simulink model "DiRe"  (Simulink 8.5)
settings: Solver=ode23t  SolverMode=SingleTasking  StartTime=0.0  StopTime=0.08  FixedStep=1e-5  MaxStep=0.7e-4  RelTol=1e-3  AbsTol=1e-2
libraries: powerlib x40, powerlib_extras x4
settings Model: Creator=azadpour  LastModifiedBy=PC
settings DataIOCC: LimitDataPoints=off
settings OptimizationCC: BlockReduction=off  BooleanDataType=off  InitFltsAndDblsToZero=on
settings DebuggingCC: SaveWithParameterizedLinksMsg=none  SignalResolutionControl=TryResolveAllWithWarning  MultiTaskDSMMsg=warning  MultiTaskCondExecSysMsg=none  FcnCallInpInsideContextMsg=UseLocalSettings
settings HardwareCC: TargetUnknown=on
settings GRTTargetCC: TargetFcnLib=ansi_tfl_tmw.mat

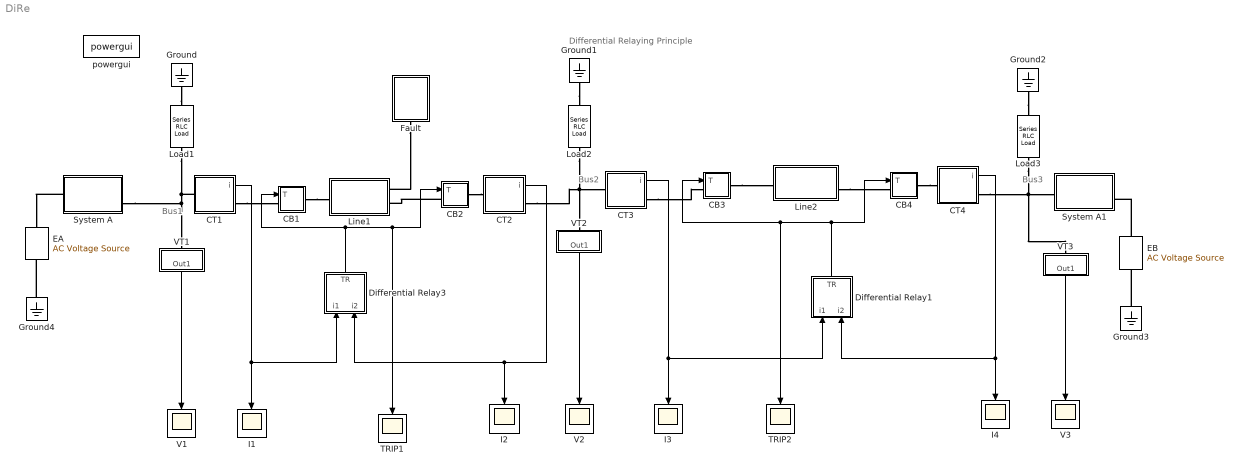
== system DiRe ==
  note: Differential Relaying Principle
  note: Bus3
  note: Bus2
  note: Bus1
  CB1 : Subsystem  mask(CB){t_op=15}
      mask prompts: t_op "Operating time [ms]"
      mask Display: disp('CB')
  CB2 : Subsystem  mask(CB){t_op=25}
      mask prompts: t_op "Operating time [ms]"
      mask Display: disp('CB')
  CB3 : Subsystem  mask(CB){t_op=18}
      mask prompts: t_op "Operating time [ms]"
      mask Display: disp('CB')
  CB4 : Subsystem  mask(CB){t_op=21}
      mask prompts: t_op "Operating time [ms]"
      mask Display: disp('CB')
  CT1 : Subsystem  mask(CT){Prim=2000, Sec=4.5}
      mask prompts: Prim "Primary Current [A]"; Sec "Secondary Current [A]"
      mask Display: disp('CT')
  CT2 : Subsystem  mask(CT){Prim=2000, Sec=1}
      mask prompts: Prim "Primary Current [A]"; Sec "Secondary Current [A]"
      mask Display: disp('CT')
  CT3 : Subsystem  mask(CT){Prim=2000, Sec=5}
      mask prompts: Prim "Primary Current [A]"; Sec "Secondary Current [A]"
      mask Display: disp('CT')
  CT4 : Subsystem  mask(CT){Prim=2000, Sec=5}
      mask prompts: Prim "Primary Current [A]"; Sec "Secondary Current [A]"
      mask Display: disp('CT')
  Differential Relay1 : Subsystem
  Differential Relay3 : Subsystem
  EA : powerlib/Electrical Sources/AC Voltage Source  Amplitude=158000  Phase=0  Frequency=60  SampleTime=0  Measurements=None
  EB : powerlib/Electrical Sources/AC Voltage Source  Amplitude=145000  Phase=-15  Frequency=60  SampleTime=0  Measurements=None
  Fault : Subsystem  mask(Fault){RF=152, tf=0.02}
      mask prompts: RF "Resistance [ohm]"; tf "Time [sec]"
      mask Display: plot(0,0,100,100,[44,47,56,38,50],[23,8,64,44,97],[56,47],[25,8])
  Ground{,1..4} (5 alike) : powerlib/Elements/Ground  LConnTagsString=a
  I{1..4} (4 alike) : Scope
      I1 settings: TickLabels=on  YMin=-20  YMax=30
      I2 settings: TickLabels=on  TimeRange=0.08  YMin=-20  YMax=30
      I3 settings: TickLabels=on  YMin=-10  YMax=20
      I4 settings: TickLabels=on  YMin=-10  YMax=20
  Line1 : Subsystem  mask(Simple Line){R=2, X=20, p=0.5}
      mask prompts: R "Resistance [ohm]"; X "Reactance [ohm]"; p "Fault location [pu]"
      mask init:
      | R1=R*p; R2=R*(1-p);
      | L1=X*p/(2*pi*60);L2=X*(1-p)/(2*pi*60);
  Line2 : Subsystem  mask(Simple Line){R=2, X=20, p=0.2}
      mask prompts: R "Resistance [ohm]"; X "Reactance [ohm]"; p "Fault location [pu]"
      mask init:
      | R1=R*p; R2=R*(1-p);
      | L1=X*p/(2*pi*60);L2=X*(1-p)/(2*pi*60);
  Load1 : powerlib/Elements/Series RLC Load  LConnTagsString=a  RConnTagsString=__new0  NominalVoltage=138e3  NominalFrequency=60  ActivePower=100e6  InductivePower=30e6  CapacitivePower=0  Setx0=off  InitialVoltage=0  SetiL0=off  InitialCurrent=0  Measurements=None
  Load2 : powerlib/Elements/Series RLC Load  LConnTagsString=a  RConnTagsString=__new0  NominalVoltage=138e3  NominalFrequency=60  ActivePower=100e6  InductivePower=30e6  CapacitivePower=0  Setx0=off  InitialVoltage=0  SetiL0=off  InitialCurrent=0  Measurements=None
  Load3 : powerlib/Elements/Series RLC Load  LConnTagsString=a  RConnTagsString=__new0  NominalVoltage=138e3  NominalFrequency=60  ActivePower=100e6  InductivePower=30e6  CapacitivePower=0  Setx0=off  InitialVoltage=0  SetiL0=off  InitialCurrent=0  Measurements=None
  System A : Subsystem  mask(Simple Line){R=1, X=10, p=0.5}
      mask prompts: R "Resistance [ohm]"; X "Reactance [ohm]"; p "Fault location [pu]"
      mask init:
      | R1=R*p; R2=R*(1-p);
      | L1=X*p/(2*pi*60);L2=X*(1-p)/(2*pi*60);
  System A1 : Subsystem  mask(Simple Line){R=1, X=10, p=0.5}
      mask prompts: R "Resistance [ohm]"; X "Reactance [ohm]"; p "Fault location [pu]"
      mask init:
      | R1=R*p; R2=R*(1-p);
      | L1=X*p/(2*pi*60);L2=X*(1-p)/(2*pi*60);
  TRIP1 : Scope
      settings: TickLabels=on  YMin=-1  YMax=2
  TRIP2 : Scope
      settings: TickLabels=on  YMin=-1  YMax=1
  V1 : Scope
      settings: TickLabels=on  YMin=-175000  YMax=175000
  V2 : Scope
      settings: TickLabels=on  YMin=-15000  YMax=15000
  V3 : Scope
      settings: TickLabels=on  YMin=-125000  YMax=125000
  VT1 : Subsystem  mask(VT){vol1=138, vol2=100}
      mask prompts: vol1 "Primary voltage [kV]"; vol2 "Secondary voltage [V]"
      mask Display: disp('VT')
  VT2 : Subsystem  mask(VT){vol1=138, vol2=100}
      mask prompts: vol1 "Primary voltage [kV]"; vol2 "Secondary voltage [V]"
      mask Display: disp('VT')
  VT3 : Subsystem  mask(VT){vol1=138, vol2=100}
      mask prompts: vol1 "Primary voltage [kV]"; vol2 "Secondary voltage [V]"
      mask Display: disp('VT')
  powergui : powerlib/powergui  SimulationMode=Continuous  SolverType=Tustin/Backward Euler (TBE)  SampleTime=0  frequency=60  SPID=off  DisableSnubberDevices=off  DisableRonSwitches=off  DisableVfSwitches=off  SwTol=0  DisplayEquations=off  Interpol=off  methode=off  Ts=0  FunctionMessages=off  echomessages=off  HookPort=off  EnableUseOfTLC=off  x0status=blocks  frequencyindice=60  Pbase=100e6  ErrMax=1e-4  Iterations=50  UnitsV=kV  UnitsW=MW  buscounter=0  RestoreLinks=warning  ResistiveCurrentMeasurement=off  Frange=[0:2:500]  Ylog=off  Xlog=on  ShowGrid=off  save=off  variable=ZData  ZoomFFT=on  StartTime=0.0  cycles=1  DisplayStyle=1  fundamental=60  FreqAxis=off  MaxFrequency=1000  frequencyindicesteady=1  RmsSteady=1  display=off
  wires:
  VT2/1(Out1) -> V2/1
  Differential Relay1/1(TR) -> CB3/1(T), TRIP2/1, CB4/1(T)
  VT1/1(Out1) -> V1/1
  CT1/1(i) -> Differential Relay3/1(i1), I1/1
  Differential Relay3/1(TR) -> CB2/1(T), TRIP1/1, CB1/1(T)
  CT3/1(i) -> I3/1, Differential Relay1/1(i1)
  CT2/1(i) -> Differential Relay3/2(i2), I2/1
  VT3/1(Out1) -> V3/1
  CT4/1(i) -> I4/1, Differential Relay1/2(i2)
  connections:
  Ground4/LConn1 -- EA/LConn1
  System A/LConn1 -- EA/RConn1
  CT1/LConn1 -- Load1/RConn1 -- VT1/LConn1 -- System A/RConn2
  Ground/LConn1 -- Load1/LConn1
  CB2/LConn1 -- Line1/RConn2
  CB1/RConn1 -- Line1/LConn1
  CT1/RConn1 -- CB1/LConn1
  CT3/RConn1 -- CB3/LConn1
  CB2/RConn1 -- CT2/LConn1
  Ground1/LConn1 -- Load2/LConn1
  CB3/RConn1 -- Line2/LConn1
  Load2/RConn1 -- VT2/LConn1 -- CT3/LConn1 -- CT2/RConn1
  Load3/RConn1 -- VT3/LConn1 -- System A1/LConn1 -- CT4/RConn1
  EB/RConn1 -- System A1/RConn2
  Ground3/LConn1 -- EB/LConn1
  CB4/RConn1 -- CT4/LConn1
  Ground2/LConn1 -- Load3/LConn1
  Line2/RConn2 -- CB4/LConn1
  Fault/LConn1 -- Line1/RConn1

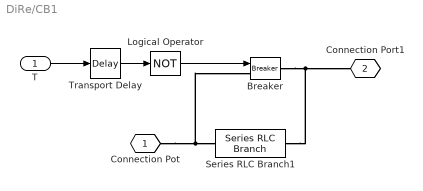
== system DiRe/CB1 ==
  T : Inport
  Breaker : powerlib/Elements/Breaker  Tag=PoWeRsYsTeMbLoCk  InitialState=1  SwitchingTimes="[ 1/60  5/60 ]"  External=on  BreakerResistance=0.01  SnubberResistance=1e6  SnubberCapacitance=inf  Measurements=None  MoreParameters=off  NoBreakLoop=off
  Logical Operator : Logic  Operator=NOT  Inputs=1
  Series RLC Branch1 : powerlib/Elements/Series RLC Branch  LConnTagsString=__new0  RConnTagsString=__new0  BranchType=R  Resistance=10000  Inductance=1.0  SetiL0=off  InitialCurrent=0  Capacitance=1.0  Setx0=off  InitialVoltage=0  Measurements=None
  Transport Delay : TransportDelay  DelayTime=t_op/1000
  Connection Pot : PMIOPort  Tag=PMCPort  Port=1  Side=Left
  Connection Port1 : PMIOPort  Tag=PMCPort  Port=2  Side=Right
  wires:
  T/1 -> Transport Delay/1
  Transport Delay/1 -> Logical Operator/1
  Logical Operator/1 -> Breaker/1
  connections:
  Connection Pot/RConn1 -- Series RLC Branch1/LConn1 -- Breaker/LConn1
  Breaker/RConn1 -- Connection Port1/RConn1 -- Series RLC Branch1/RConn1

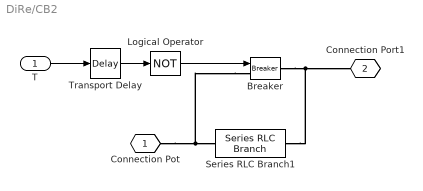
== system DiRe/CB2 ==
  T : Inport
  Breaker : powerlib/Elements/Breaker  Tag=PoWeRsYsTeMbLoCk  InitialState=1  SwitchingTimes="[ 1/60  5/60 ]"  External=on  BreakerResistance=0.01  SnubberResistance=1e6  SnubberCapacitance=inf  Measurements=None  MoreParameters=off  NoBreakLoop=off
  Logical Operator : Logic  Operator=NOT  Inputs=1
  Series RLC Branch1 : powerlib/Elements/Series RLC Branch  LConnTagsString=__new0  RConnTagsString=__new0  BranchType=R  Resistance=10000  Inductance=1e-3  SetiL0=off  InitialCurrent=0  Capacitance=1e-6  Setx0=off  InitialVoltage=0  Measurements=None
  Transport Delay : TransportDelay  DelayTime=t_op/1000
  Connection Pot : PMIOPort  Tag=PMCPort  Port=1  Side=Left
  Connection Port1 : PMIOPort  Tag=PMCPort  Port=2  Side=Right
  wires:
  Logical Operator/1 -> Breaker/1
  Transport Delay/1 -> Logical Operator/1
  T/1 -> Transport Delay/1
  connections:
  Series RLC Branch1/RConn1 -- Connection Port1/RConn1 -- Breaker/RConn1
  Breaker/LConn1 -- Series RLC Branch1/LConn1 -- Connection Pot/RConn1

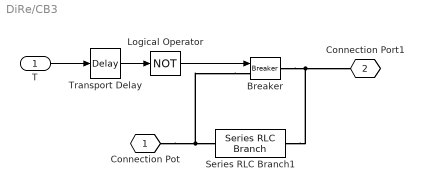
== system DiRe/CB3 ==
  T : Inport
  Breaker : powerlib/Elements/Breaker  Tag=PoWeRsYsTeMbLoCk  InitialState=1  SwitchingTimes="[ 1/60  5/60 ]"  External=on  BreakerResistance=0.01  SnubberResistance=1e6  SnubberCapacitance=inf  Measurements=None  MoreParameters=off  NoBreakLoop=off
  Logical Operator : Logic  Operator=NOT  Inputs=1
  Series RLC Branch1 : powerlib/Elements/Series RLC Branch  LConnTagsString=__new0  RConnTagsString=__new0  BranchType=R  Resistance=10000  Inductance=1e-3  SetiL0=off  InitialCurrent=0  Capacitance=1e-6  Setx0=off  InitialVoltage=0  Measurements=None
  Transport Delay : TransportDelay  DelayTime=t_op/1000
  Connection Pot : PMIOPort  Tag=PMCPort  Port=1  Side=Left
  Connection Port1 : PMIOPort  Tag=PMCPort  Port=2  Side=Right
  wires:
  Logical Operator/1 -> Breaker/1
  Transport Delay/1 -> Logical Operator/1
  T/1 -> Transport Delay/1
  connections:
  Series RLC Branch1/RConn1 -- Connection Port1/RConn1 -- Breaker/RConn1
  Breaker/LConn1 -- Series RLC Branch1/LConn1 -- Connection Pot/RConn1

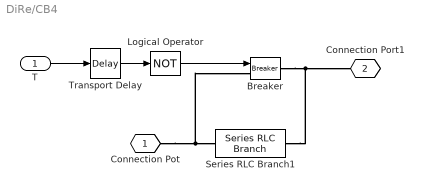
== system DiRe/CB4 ==
  T : Inport
  Breaker : powerlib/Elements/Breaker  Tag=PoWeRsYsTeMbLoCk  InitialState=1  SwitchingTimes="[ 1/60  5/60 ]"  External=on  BreakerResistance=0.01  SnubberResistance=1e6  SnubberCapacitance=inf  Measurements=None  MoreParameters=off  NoBreakLoop=off
  Logical Operator : Logic  Operator=NOT  Inputs=1
  Series RLC Branch1 : powerlib/Elements/Series RLC Branch  LConnTagsString=__new0  RConnTagsString=__new0  BranchType=R  Resistance=10000  Inductance=1e-3  SetiL0=off  InitialCurrent=0  Capacitance=1e-6  Setx0=off  InitialVoltage=0  Measurements=None
  Transport Delay : TransportDelay  DelayTime=t_op/1000
  Connection Pot : PMIOPort  Tag=PMCPort  Port=1  Side=Left
  Connection Port1 : PMIOPort  Tag=PMCPort  Port=2  Side=Right
  wires:
  T/1 -> Transport Delay/1
  Transport Delay/1 -> Logical Operator/1
  Logical Operator/1 -> Breaker/1
  connections:
  Connection Pot/RConn1 -- Series RLC Branch1/LConn1 -- Breaker/LConn1
  Breaker/RConn1 -- Connection Port1/RConn1 -- Series RLC Branch1/RConn1

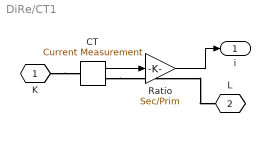
== system DiRe/CT1 ==
  CT : powerlib/Measurements/Current Measurement  PhasorSimulation=off  OutputType=Complex  PSBequivalent=0
  Ratio : Gain  Gain=Sec/Prim  SaturateOnIntegerOverflow=on  OutDataTypeStr=Inherit: Same as input  ParamDataTypeStr=Inherit: Same as input
  K : PMIOPort  Tag=PMCPort  Port=1  Side=Left
  L : PMIOPort  Tag=PMCPort  Port=2  Side=Right
  i : Outport  InitialOutput=0
  wires:
  CT/1 -> Ratio/1
  Ratio/1 -> i/1
  connections:
  K/RConn1 -- CT/LConn1
  CT/RConn1 -- L/RConn1

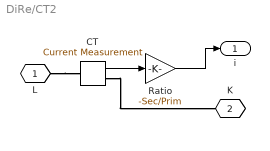
== system DiRe/CT2 ==
  CT : powerlib/Measurements/Current Measurement  PhasorSimulation=off  OutputType=Complex  PSBequivalent=0
  Ratio : Gain  Gain=-Sec/Prim  SaturateOnIntegerOverflow=on  OutDataTypeStr=Inherit: Same as input  ParamDataTypeStr=Inherit: Same as input
  L : PMIOPort  Tag=PMCPort  Port=1  Side=Left
  K : PMIOPort  Tag=PMCPort  Port=2  Side=Right
  i : Outport  InitialOutput=0
  wires:
  Ratio/1 -> i/1
  CT/1 -> Ratio/1
  connections:
  CT/RConn1 -- K/RConn1
  L/RConn1 -- CT/LConn1

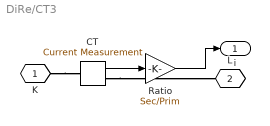
== system DiRe/CT3 ==
  CT : powerlib/Measurements/Current Measurement  PhasorSimulation=off  OutputType=Complex  PSBequivalent=0
  Ratio : Gain  Gain=Sec/Prim  SaturateOnIntegerOverflow=on  OutDataTypeStr=Inherit: Same as input  ParamDataTypeStr=Inherit: Same as input
  K : PMIOPort  Tag=PMCPort  Port=1  Side=Left
  L : PMIOPort  Tag=PMCPort  Port=2  Side=Right
  i : Outport  InitialOutput=0
  wires:
  Ratio/1 -> i/1
  CT/1 -> Ratio/1
  connections:
  CT/RConn1 -- L/RConn1
  K/RConn1 -- CT/LConn1

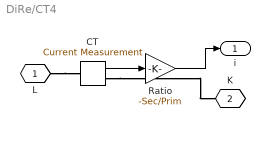
== system DiRe/CT4 ==
  CT : powerlib/Measurements/Current Measurement  PhasorSimulation=off  OutputType=Complex  PSBequivalent=0
  Ratio : Gain  Gain=-Sec/Prim  SaturateOnIntegerOverflow=on  OutDataTypeStr=Inherit: Same as input  ParamDataTypeStr=Inherit: Same as input
  L : PMIOPort  Tag=PMCPort  Port=1  Side=Left
  K : PMIOPort  Tag=PMCPort  Port=2  Side=Right
  i : Outport  InitialOutput=0
  wires:
  CT/1 -> Ratio/1
  Ratio/1 -> i/1
  connections:
  L/RConn1 -- CT/LConn1
  CT/RConn1 -- K/RConn1

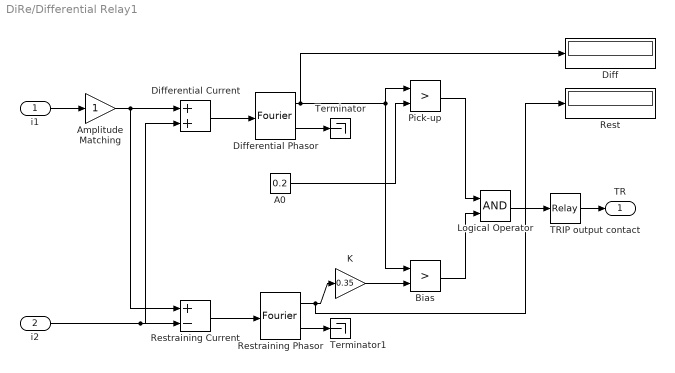
== system DiRe/Differential Relay1 ==
  i1 : Inport
  i2 : Inport  Port=2
  A0 : Constant  Value=0.2
  Amplitude Matching : Gain  SaturateOnIntegerOverflow=on  OutDataTypeStr=Inherit: Same as input  ParamDataTypeStr=Inherit: Same as input
  Bias : RelationalOperator  Operator=>  InputSameDT=on
  Diff : Display
  Differential Current : Sum  SaturateOnIntegerOverflow=on  InputSameDT=on  OutDataTypeStr=Inherit: Same as first input
  Differential Phasor : powerlib_extras/Measurements/Fourier  f1=60  n=1
  K : Gain  Gain=0.35  SaturateOnIntegerOverflow=on  OutDataTypeStr=Inherit: Same as input  ParamDataTypeStr=Inherit: Same as input
  Logical Operator : Logic
  Pick-up : RelationalOperator  Operator=>  InputSameDT=on
  Rest : Display
  Restraining Current : Sum  Inputs=+-  SaturateOnIntegerOverflow=on  InputSameDT=on  OutDataTypeStr=Inherit: Same as first input
  Restraining Phasor : powerlib_extras/Measurements/Fourier  f1=60  n=1
  TRIP output contact : Relay  OnSwitchValue=0.9999  OffSwitchValue=-1
  Terminator : Terminator
  Terminator1 : Terminator
  TR : Outport  InitialOutput=0
  wires:
  i1/1 -> Amplitude Matching/1
  Amplitude Matching/1 -> Differential Current/1, Restraining Current/1
  Differential Phasor/2 -> Terminator/1
  i2/1 -> Differential Current/2, Restraining Current/2
  Restraining Current/1 -> Restraining Phasor/1
  Restraining Phasor/2 -> Terminator1/1
  K/1 -> Bias/2
  A0/1 -> Pick-up/2
  Differential Current/1 -> Differential Phasor/1
  Bias/1 -> Logical Operator/2
  Pick-up/1 -> Logical Operator/1
  TRIP output contact/1 -> TR/1
  Logical Operator/1 -> TRIP output contact/1
  Differential Phasor/1 -> Bias/1, Pick-up/1, Diff/1
  Restraining Phasor/1 -> K/1, Rest/1

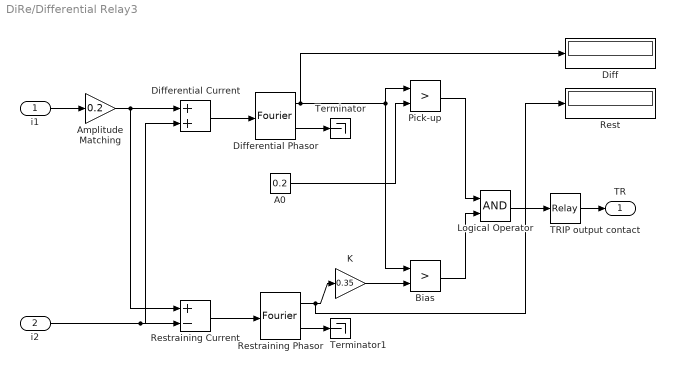
== system DiRe/Differential Relay3 ==
  i1 : Inport
  i2 : Inport  Port=2
  A0 : Constant  Value=0.2
  Amplitude Matching : Gain  Gain=0.2  SaturateOnIntegerOverflow=on  OutDataTypeStr=Inherit: Same as input  ParamDataTypeStr=Inherit: Same as input
  Bias : RelationalOperator  Operator=>  InputSameDT=on
  Diff : Display
  Differential Current : Sum  SaturateOnIntegerOverflow=on  InputSameDT=on  OutDataTypeStr=Inherit: Same as first input
  Differential Phasor : powerlib_extras/Measurements/Fourier  f1=60  n=1
  K : Gain  Gain=0.35  SaturateOnIntegerOverflow=on  OutDataTypeStr=Inherit: Same as input  ParamDataTypeStr=Inherit: Same as input
  Logical Operator : Logic
  Pick-up : RelationalOperator  Operator=>  InputSameDT=on
  Rest : Display
  Restraining Current : Sum  Inputs=+-  SaturateOnIntegerOverflow=on  InputSameDT=on  OutDataTypeStr=Inherit: Same as first input
  Restraining Phasor : powerlib_extras/Measurements/Fourier  f1=60  n=1
  TRIP output contact : Relay  OnSwitchValue=0.9999  OffSwitchValue=-1
  Terminator : Terminator
  Terminator1 : Terminator
  TR : Outport  InitialOutput=0
  wires:
  Restraining Phasor/1 -> Rest/1, K/1
  Differential Phasor/1 -> Diff/1, Pick-up/1, Bias/1
  Logical Operator/1 -> TRIP output contact/1
  TRIP output contact/1 -> TR/1
  Pick-up/1 -> Logical Operator/1
  Bias/1 -> Logical Operator/2
  Differential Current/1 -> Differential Phasor/1
  A0/1 -> Pick-up/2
  K/1 -> Bias/2
  Restraining Phasor/2 -> Terminator1/1
  Restraining Current/1 -> Restraining Phasor/1
  i2/1 -> Restraining Current/2, Differential Current/2
  Differential Phasor/2 -> Terminator/1
  Amplitude Matching/1 -> Restraining Current/1, Differential Current/1
  i1/1 -> Amplitude Matching/1

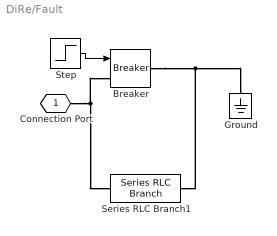
== system DiRe/Fault ==
  Breaker : powerlib/Elements/Breaker  Tag=PoWeRsYsTeMbLoCk  InitialState=0  SwitchingTimes="[ 1/60  5/60 ]"  External=on  BreakerResistance=0.01  SnubberResistance=1e6  SnubberCapacitance=inf  Measurements=None  MoreParameters=off  NoBreakLoop=off
  Ground : powerlib/Elements/Ground  LConnTagsString=a
  Series RLC Branch1 : powerlib/Elements/Series RLC Branch  LConnTagsString=__new0  RConnTagsString=__new0  BranchType=RLC  Resistance=1  Inductance=1e-3  SetiL0=off  InitialCurrent=0  Capacitance=1e-6  Setx0=off  InitialVoltage=0  Measurements=None
  Step : Step  Time=tf
  Connection Port : PMIOPort  Tag=PMCPort  Port=1  Side=Left
  wires:
  Step/1 -> Breaker/1
  connections:
  Breaker/RConn1 -- Ground/LConn1 -- Series RLC Branch1/RConn1
  Connection Port/RConn1 -- Breaker/LConn1 -- Series RLC Branch1/LConn1

== system DiRe/Line1 ==
  Series RLC Branch : powerlib/Elements/Series RLC Branch  LConnTagsString=__new0  RConnTagsString=__new0  BranchType=RL  Resistance=R1  Inductance=L1  SetiL0=off  InitialCurrent=0  Capacitance=1.0  Setx0=off  InitialVoltage=0  Measurements=None
  Series RLC Branch1 : powerlib/Elements/Series RLC Branch  LConnTagsString=__new0  RConnTagsString=__new0  BranchType=RL  Resistance=R2  Inductance=L2  SetiL0=off  InitialCurrent=0  Capacitance=1.0  Setx0=off  InitialVoltage=0  Measurements=None
  A : PMIOPort  Tag=PMCPort  Port=1  Side=Left
  Fault : PMIOPort  Tag=PMCPort  Port=2  Side=Right
  B : PMIOPort  Tag=PMCPort  Port=3  Side=Right
  connections:
  A/RConn1 -- Series RLC Branch/LConn1
  Fault/RConn1 -- Series RLC Branch/RConn1 -- Series RLC Branch1/LConn1
  Series RLC Branch1/RConn1 -- B/RConn1

== system DiRe/Line2 ==
  Series RLC Branch : powerlib/Elements/Series RLC Branch  LConnTagsString=__new0  RConnTagsString=__new0  BranchType=RL  Resistance=R1  Inductance=L1  SetiL0=off  InitialCurrent=0  Capacitance=1.0  Setx0=off  InitialVoltage=0  Measurements=None
  Series RLC Branch1 : powerlib/Elements/Series RLC Branch  LConnTagsString=__new0  RConnTagsString=__new0  BranchType=RL  Resistance=R2  Inductance=L2  SetiL0=off  InitialCurrent=0  Capacitance=1.0  Setx0=off  InitialVoltage=0  Measurements=None
  A : PMIOPort  Tag=PMCPort  Port=1  Side=Left
  Fault : PMIOPort  Tag=PMCPort  Port=2  Side=Right
  B : PMIOPort  Tag=PMCPort  Port=3  Side=Right
  connections:
  Series RLC Branch1/RConn1 -- B/RConn1
  Series RLC Branch/RConn1 -- Fault/RConn1 -- Series RLC Branch1/LConn1
  A/RConn1 -- Series RLC Branch/LConn1

== system DiRe/System A ==
  Series RLC Branch : powerlib/Elements/Series RLC Branch  LConnTagsString=__new0  RConnTagsString=__new0  BranchType=RL  Resistance=R1  Inductance=L1  SetiL0=off  InitialCurrent=0  Capacitance=1.0  Setx0=off  InitialVoltage=0  Measurements=None
  Series RLC Branch1 : powerlib/Elements/Series RLC Branch  LConnTagsString=__new0  RConnTagsString=__new0  BranchType=RL  Resistance=R2  Inductance=L2  SetiL0=off  InitialCurrent=0  Capacitance=1.0  Setx0=off  InitialVoltage=0  Measurements=None
  A : PMIOPort  Tag=PMCPort  Port=1  Side=Left
  Fault : PMIOPort  Tag=PMCPort  Port=2  Side=Right
  B : PMIOPort  Tag=PMCPort  Port=3  Side=Right
  connections:
  Series RLC Branch1/RConn1 -- B/RConn1
  Series RLC Branch/RConn1 -- Fault/RConn1 -- Series RLC Branch1/LConn1
  A/RConn1 -- Series RLC Branch/LConn1

== system DiRe/System A1 ==
  Series RLC Branch : powerlib/Elements/Series RLC Branch  LConnTagsString=__new0  RConnTagsString=__new0  BranchType=RL  Resistance=R1  Inductance=L1  SetiL0=off  InitialCurrent=0  Capacitance=1.0  Setx0=off  InitialVoltage=0  Measurements=None
  Series RLC Branch1 : powerlib/Elements/Series RLC Branch  LConnTagsString=__new0  RConnTagsString=__new0  BranchType=RL  Resistance=R2  Inductance=L2  SetiL0=off  InitialCurrent=0  Capacitance=1.0  Setx0=off  InitialVoltage=0  Measurements=None
  A : PMIOPort  Tag=PMCPort  Port=1  Side=Left
  Fault : PMIOPort  Tag=PMCPort  Port=2  Side=Right
  B : PMIOPort  Tag=PMCPort  Port=3  Side=Right
  connections:
  Series RLC Branch1/RConn1 -- B/RConn1
  Series RLC Branch/RConn1 -- Fault/RConn1 -- Series RLC Branch1/LConn1
  A/RConn1 -- Series RLC Branch/LConn1

== system DiRe/VT1 ==
  Ground : powerlib/Elements/Ground  LConnTagsString=a
  PP : powerlib/Measurements/Voltage Measurement  Tag=PoWeRsYsTeMmEaSuReMeNt  PhasorSimulation=off  OutputType=Complex  PSBequivalent=0
  ratio : Gain  Gain=vol2/(vol1*1000)  SaturateOnIntegerOverflow=on  OutDataTypeStr=Inherit: Same as input  ParamDataTypeStr=Inherit: Same as input
  Connection Port1 : PMIOPort  Tag=PMCPort  Port=1  Side=Left
  Out1 : Outport  InitialOutput=0
  wires:
  PP/1 -> ratio/1
  ratio/1 -> Out1/1
  connections:
  Connection Port1/RConn1 -- PP/LConn1
  Ground/LConn1 -- PP/LConn2

== system DiRe/VT2 ==
  Ground : powerlib/Elements/Ground  LConnTagsString=a
  PP : powerlib/Measurements/Voltage Measurement  Tag=PoWeRsYsTeMmEaSuReMeNt  PhasorSimulation=off  OutputType=Complex  PSBequivalent=0
  ratio : Gain  Gain=vol2/(vol1*1000)  SaturateOnIntegerOverflow=on  OutDataTypeStr=Inherit: Same as input  ParamDataTypeStr=Inherit: Same as input
  Connection Port1 : PMIOPort  Tag=PMCPort  Port=1  Side=Left
  Out1 : Outport  InitialOutput=0
  wires:
  ratio/1 -> Out1/1
  PP/1 -> ratio/1
  connections:
  Ground/LConn1 -- PP/LConn2
  Connection Port1/RConn1 -- PP/LConn1

== system DiRe/VT3 ==
  Ground : powerlib/Elements/Ground  LConnTagsString=a
  PP : powerlib/Measurements/Voltage Measurement  Tag=PoWeRsYsTeMmEaSuReMeNt  PhasorSimulation=off  OutputType=Complex  PSBequivalent=0
  ratio : Gain  Gain=vol2/(vol1*1000)  SaturateOnIntegerOverflow=on  OutDataTypeStr=Inherit: Same as input  ParamDataTypeStr=Inherit: Same as input
  Connection Port1 : PMIOPort  Tag=PMCPort  Port=1  Side=Left
  Out1 : Outport  InitialOutput=0
  wires:
  PP/1 -> ratio/1
  ratio/1 -> Out1/1
  connections:
  Connection Port1/RConn1 -- PP/LConn1
  Ground/LConn1 -- PP/LConn2
